simulink model "mydct"  (R2018b)
settings: Solver=VariableStepAuto  StartTime=0.0  StopTime=0  RelTol=1e-3
libraries: visionsources x1
settings Model: Creator=DSP-36  LastModifiedBy=DSP-36

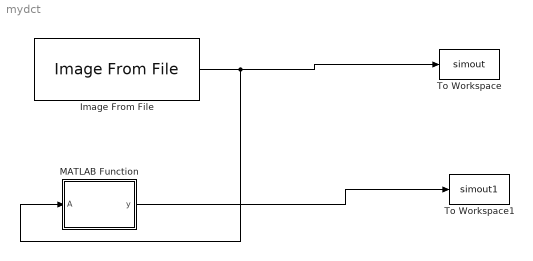
== system mydct ==
  Image From File : visionsources/Image From File  Tag=vipblks_nd  FileName=C:\Users\DSP-36\Desktop\17ucc038\cameraman.tif  imagePorts=One multidimensional signal  Ts=inf  ImageDataType=Inherit from input image  Signed=on  WordLength=16  sdImageDataType=uint(8)  FractionLengthMode=User-defined  FractionLength=15  OutPortLabels=R|G|B
      settings: SourceProductName=Computer Vision System Toolbox
  MATLAB Function : MATLAB Function  TreatAsAtomicUnit=on
  To Workspace : ToWorkspace  VariableName=simout  SampleTime=-1
  To Workspace1 : ToWorkspace  VariableName=simout1  SampleTime=-1
  wires:
  Image From File/1 -> MATLAB Function/1(A), To Workspace/1
  MATLAB Function/1(y) -> To Workspace1/1

== matlab function mydct/MATLAB Function ==
  data: A input; y output
function y = mydct(A)
y = zeros(size(A,1));
coder.extrinsic('dct2');
coder.extrinsic('idct2');
Q = dct2(A);
Rim = [Q(1:128,1:128),zeros(128);zeros(128,256)];
y = idct2(Rim);
